simulink model "PID_final"  (R2020a)
settings: Solver=VariableStepAuto  StartTime=0.0  StopTime=10.0  RelTol=1e-3
values from neighbouring files (symbols this model uses):
  B = .1    (= 0.1)    [parameters.m]
  J = .01    (= 0.01)    [parameters.m]
  K = .01    (= 0.01)    [parameters.m]
  L = .5    (= 0.5)    [parameters.m]
  R = 1    [parameters.m]
settings Model: Creator=Maria  LastModifiedBy=Maria

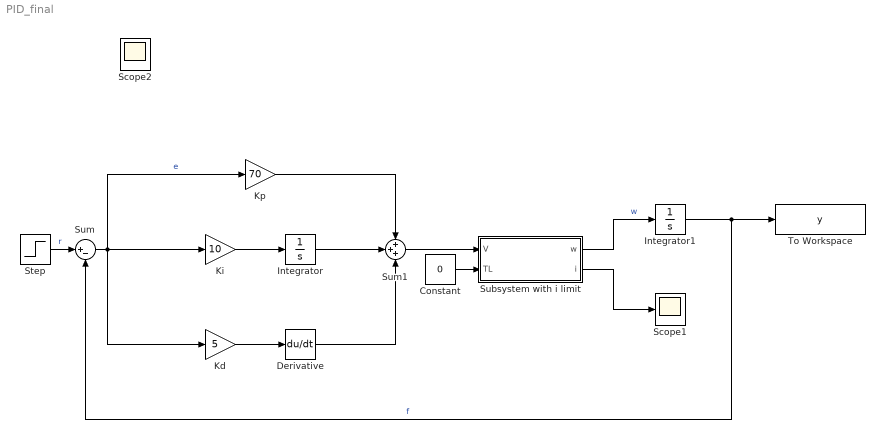
== system PID_final ==
  Constant : Constant  Value=0
  Derivative : Derivative
  Integrator : Integrator
  Integrator1 : Integrator
  Kd : Gain  Gain=5
  Ki : Gain  Gain=10
  Kp : Gain  Gain=70
  Scope1 : Scope
  Step : Step  Time=0  SampleTime=0
  Subsystem with i limit : Subsystem
  Sum : Sum  Inputs=|+-
  Sum1 : Sum  Inputs=+++
  To Workspace : ToWorkspace  VariableName=y  SaveFormat=Timeseries  SampleTime=-1
  Scope2 : Scope
  wires:
  Integrator1/1 -> To Workspace/1, Sum/2  "f"
  Step/1 -> Sum/1  "r"
  Integrator/1 -> Sum1/2
  Ki/1 -> Integrator/1
  Sum/1 -> Kd/1, Kp/1, Ki/1  "e"
  Kp/1 -> Sum1/1
  Kd/1 -> Derivative/1
  Derivative/1 -> Sum1/3
  Subsystem with i limit/1(w) -> Integrator1/1  "w"
  Sum1/1 -> Subsystem with i limit/1(V)
  Constant/1 -> Subsystem with i limit/2(TL)
  Subsystem with i limit/2(i) -> Scope1/1

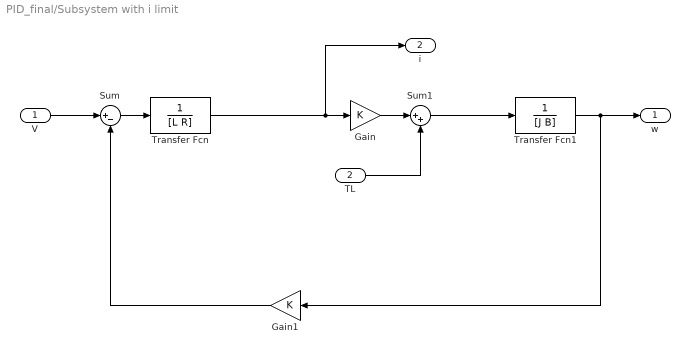
== system PID_final/Subsystem with i limit ==
  V : Inport
  TL : Inport  Port=2
  Gain : Gain  Gain=K
  Gain1 : Gain  Gain=K
  Sum : Sum  Inputs=|+-
  Sum1 : Sum  Inputs=|++
  Transfer Fcn : TransferFcn  Denominator=[L R]
  Transfer Fcn1 : TransferFcn  Denominator=[J B]
  w : Outport  VectorParamsAs1DForOutWhenUnconnected=off
  i : Outport  Port=2  VectorParamsAs1DForOutWhenUnconnected=off
  wires:
  Transfer Fcn1/1 -> w/1, Gain1/1
  Gain1/1 -> Sum/2
  V/1 -> Sum/1
  Sum/1 -> Transfer Fcn/1
  Gain/1 -> Sum1/1
  Sum1/1 -> Transfer Fcn1/1
  TL/1 -> Sum1/2
  Transfer Fcn/1 -> Gain/1, i/1
